simulink model "heli_ss"  (Simulink 8.7)
settings: Solver=VariableStepAuto  StartTime=0.0  StopTime=40.0  RelTol=1e-3
settings Model: Creator=soonchee  LastModifiedBy=soonchee
settings DataIOCC: LimitDataPoints=off  SaveFormat=Dataset
settings DebuggingCC: UnderspecifiedInitializationDetection=Simplified  MergeDetectMultiDrivingBlocksExec=error
settings HardwareCC: ProdBitPerPointer=64  ProdLargestAtomicFloat=Float  ProdIntDivRoundTo=Zero  ProdEndianess=LittleEndian  ProdWordSize=64  ProdHWDeviceType=Intel->x86-64 (Windows64)
settings ModelReferenceCC: PropagateSignalLabelsOutOfModel=on
settings ConfigComp: CovModelRefEnable=off

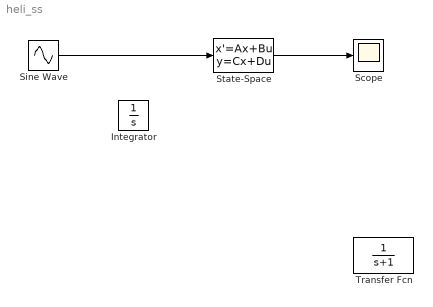
== system heli_ss ==
  Integrator : Integrator
  Scope : Scope
  Sine Wave : Sin  Amplitude=0.1  Frequency=10  SampleTime=0
  State-Space : StateSpace  A=[-0.4 0 -0.01; 1 0 0; -1.4 9.8 -0.02]  B=[6.3; 0; 9.8]  C=[0 0 1]  D=0  X0=0
  Transfer Fcn : TransferFcn  Denominator=[1 1]
  wires:
  Sine Wave/1 -> State-Space/1
  State-Space/1 -> Scope/1
